simulink library "inverter_model"  (R2025b)
settings: Solver=VariableStepAuto  StartTime=0.0  StopTime=10.0  RelTol=1e-3
settings Model: Creator=jessi  LastModifiedBy=jessi

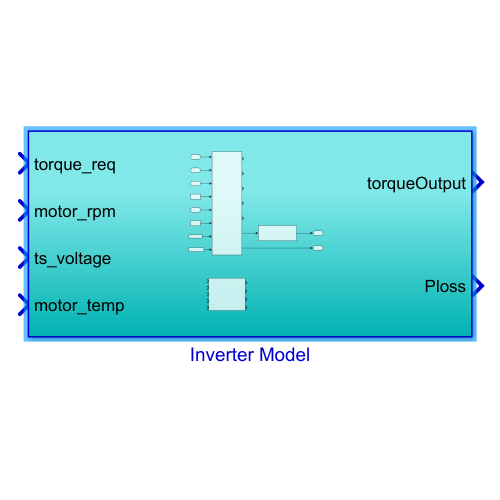
[thumbnail: Simulink's stored preview of the top-level diagram]
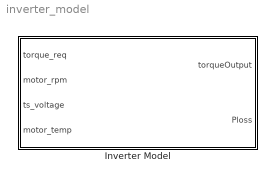
== system inverter_model ==
  Inverter Model : Subsystem

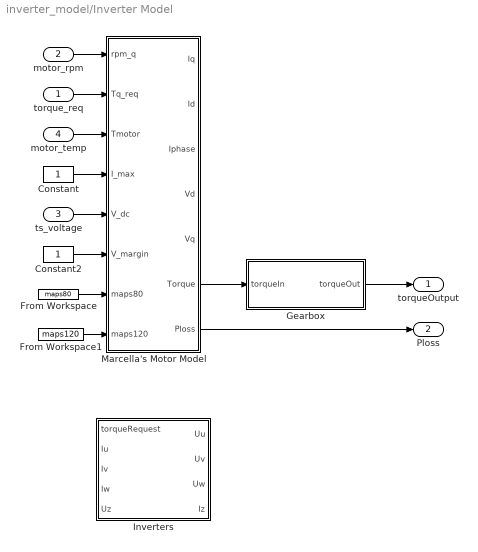
== system inverter_model/Inverter Model ==
  torque_req : Inport  Unit=N*m
  motor_rpm : Inport  Port=2  Unit=rpm
  ts_voltage : Inport  Port=3  Unit=V
  motor_temp : Inport  Port=4
  Constant : Constant
  Constant2 : Constant
  From Workspace : FromWorkspace  VariableName=maps80
  From Workspace1 : FromWorkspace  VariableName=maps120
  Gearbox : Subsystem
  Inverters : Subsystem
  Marcella's Motor Model : MATLAB Function  TreatAsAtomicUnit=on
  torqueOutput : Outport  Unit=N*m
  Ploss : Outport  Port=2  Unit=A
  wires:
  torque_req/1 -> Marcella's Motor Model/2(Tq_req)
  Gearbox/1(torqueOut) -> torqueOutput/1
  From Workspace1/1 -> Marcella's Motor Model/8(maps120)
  From Workspace/1 -> Marcella's Motor Model/7(maps80)
  motor_rpm/1 -> Marcella's Motor Model/1(rpm_q)
  Marcella's Motor Model/6(Torque) -> Gearbox/1(torqueIn)
  Marcella's Motor Model/7(Ploss) -> Ploss/1
  motor_temp/1 -> Marcella's Motor Model/3(Tmotor)
  Constant/1 -> Marcella's Motor Model/4(I_max)
  Constant2/1 -> Marcella's Motor Model/6(V_margin)
  ts_voltage/1 -> Marcella's Motor Model/5(V_dc)

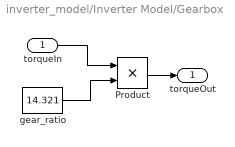
== system inverter_model/Inverter Model/Gearbox ==
  torqueIn : Inport
  Product : Product
  gear_ratio : Constant  Value=14.321
  torqueOut : Outport
  wires:
  torqueIn/1 -> Product/1
  Product/1 -> torqueOut/1
  gear_ratio/1 -> Product/2

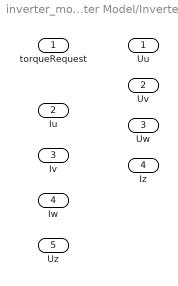
== system inverter_model/Inverter Model/Inverters ==
  torqueRequest : Inport
  Iu : Inport  Port=2
  Iv : Inport  Port=3
  Iw : Inport  Port=4
  Uz : Inport  Port=5
  Uu : Outport
  Uv : Outport  Port=2
  Uw : Outport  Port=3
  Iz : Outport  Port=4

== matlab function inverter_model/Inverter Model/Marcella's Motor Model ==
  data: rpm_q input; Tq_req input; Tmotor input; I_max input; V_dc input; V_margin input; maps80 input; maps120 input; Iq output; Id output; Iphase output; Vd output; Vq output; Torque output; Ploss output
function [Iq, Id, Iphase, Vd, Vq, Torque, Ploss]= fcn(rpm_q,Tq_req, Tmotor, I_max, V_dc, V_margin, maps80, maps120)
    limits = struct();
    limits.I_max = I_max;
    limits.V_dc = V_dc;
    limits.V_margin = V_margin;
    out = motor_map_model_function(rpm_q, Tq_req, Tmotor, maps80, maps120, limits);
    Iq = out.Iq;
    Id = out.Id;
    Iphase = out.Iphase;
    Vd = out.Vd;
    Vq = out.Vq;
    Torque = out.Torque;
    Ploss = out.Ploss;
end
